simulink model "adapt_mem"  (Simulink 7.9)
settings: Solver=ode45  StartTime=0.0  StopTime=100  RelTol=1e-3
settings Model: Creator=Floater  LastModifiedBy=jdenil
settings OptimizationCC: InlineParams=on  InitFltsAndDblsToZero=on
settings DebuggingCC: FcnCallInpInsideContextMsg=Use local settings  StrictBusMsg=Warning
settings GRTTargetCC: CombineOutputUpdateFcns=off  GRTInterface=on

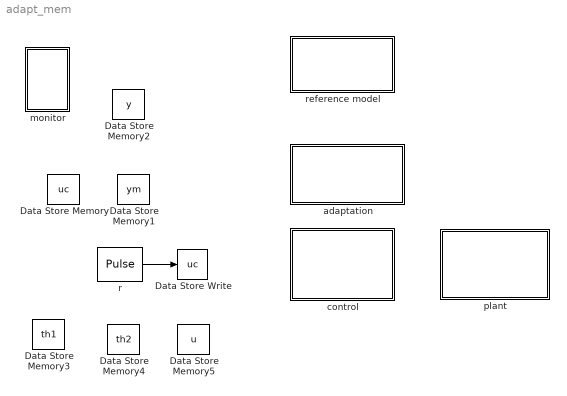
== system adapt_mem ==
  Data Store Memory : DataStoreMemory  DataStoreName=uc  ReadBeforeWriteMsg=warning  WriteAfterWriteMsg=warning  WriteAfterReadMsg=warning
  Data Store Memory1 : DataStoreMemory  DataStoreName=ym  ReadBeforeWriteMsg=warning  WriteAfterWriteMsg=warning  WriteAfterReadMsg=warning
  Data Store Memory2 : DataStoreMemory  DataStoreName=y  ReadBeforeWriteMsg=warning  WriteAfterWriteMsg=warning  WriteAfterReadMsg=warning
  Data Store Memory3 : DataStoreMemory  DataStoreName=th1  ReadBeforeWriteMsg=warning  WriteAfterWriteMsg=warning  WriteAfterReadMsg=warning
  Data Store Memory4 : DataStoreMemory  DataStoreName=th2  ReadBeforeWriteMsg=warning  WriteAfterWriteMsg=warning  WriteAfterReadMsg=warning
  Data Store Memory5 : DataStoreMemory  DataStoreName=u  ReadBeforeWriteMsg=warning  WriteAfterWriteMsg=warning  WriteAfterReadMsg=warning
  Data Store Write : DataStoreWrite  DataStoreName=uc
  adaptation : Subsystem  TreatAsAtomicUnit=on
  control : Subsystem  TreatAsAtomicUnit=on
      settings: AttributesFormatString=%<IsSubsystemVirtual>\n%<TreatAsAtomicUnit>
  monitor : Subsystem  TreatAsAtomicUnit=on
  plant : Subsystem  Priority=1  TreatAsAtomicUnit=on
  r : DiscretePulseGenerator  PulseType=Time based  Period=20  PulseWidth=50
  reference model : Subsystem  TreatAsAtomicUnit=on
      settings: AttributesFormatString=%<Priority>
  wires:
  r/1 -> Data Store Write/1

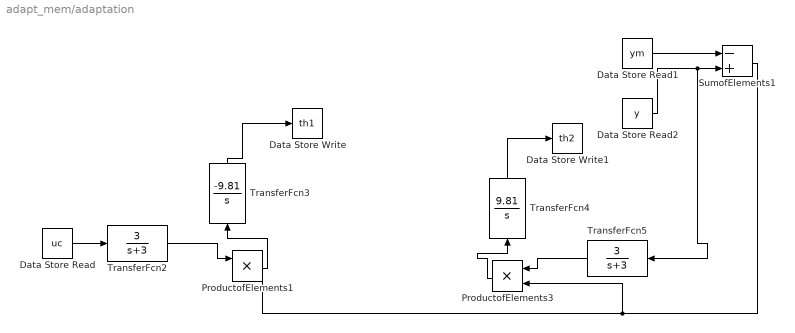
== system adapt_mem/adaptation ==
  Data Store Read : DataStoreRead  DataStoreName=uc
  Data Store Read1 : DataStoreRead  DataStoreName=ym
  Data Store Read2 : DataStoreRead  DataStoreName=y
  Data Store Write : DataStoreWrite  DataStoreName=th1
  Data Store Write1 : DataStoreWrite  DataStoreName=th2
  ProductofElements1 : Product  Inputs=**
  ProductofElements3 : Product  Inputs=**
  SumofElements1 : Sum  Inputs=-+
  TransferFcn2 : TransferFcn  Numerator=[3]  Denominator=[1 3]
  TransferFcn3 : TransferFcn  Numerator=[-9.81]  Denominator=[1 0]
  TransferFcn4 : TransferFcn  Numerator=[9.81]  Denominator=[1 0]
  TransferFcn5 : TransferFcn  Numerator=[3]  Denominator=[1 3]
  wires:
  TransferFcn2/1 -> ProductofElements1/1
  ProductofElements1/1 -> TransferFcn3/1
  TransferFcn3/1 -> Data Store Write/1
  TransferFcn4/1 -> Data Store Write1/1
  ProductofElements3/1 -> TransferFcn4/1
  TransferFcn5/1 -> ProductofElements3/1
  SumofElements1/1 -> ProductofElements1/2, ProductofElements3/2
  Data Store Read2/1 -> SumofElements1/2, TransferFcn5/1
  Data Store Read/1 -> TransferFcn2/1
  Data Store Read1/1 -> SumofElements1/1

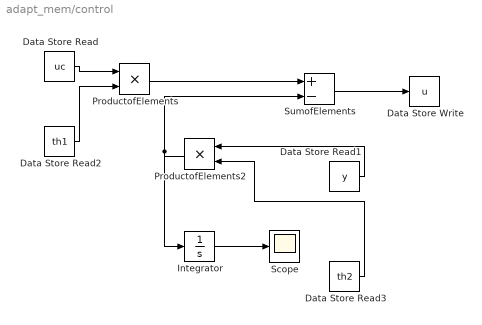
== system adapt_mem/control ==
  Data Store Read : DataStoreRead  DataStoreName=uc
  Data Store Read1 : DataStoreRead  DataStoreName=y
  Data Store Read2 : DataStoreRead  DataStoreName=th1
  Data Store Read3 : DataStoreRead  DataStoreName=th2
  Data Store Write : DataStoreWrite  DataStoreName=u
  Integrator : Integrator
  ProductofElements : Product  Inputs=**
  ProductofElements2 : Product  Inputs=**
  Scope : Scope
      settings: SaveName=ScopeData2
  SumofElements : Sum  Inputs=+-
  wires:
  ProductofElements/1 -> SumofElements/1
  ProductofElements2/1 -> Integrator/1, SumofElements/2
  Data Store Read/1 -> ProductofElements/1
  Data Store Read2/1 -> ProductofElements/2
  Data Store Read1/1 -> ProductofElements2/1
  Data Store Read3/1 -> ProductofElements2/2
  SumofElements/1 -> Data Store Write/1
  Integrator/1 -> Scope/1

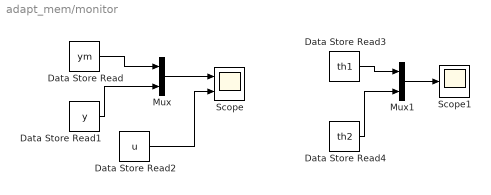
== system adapt_mem/monitor ==
  Data Store Read : DataStoreRead  DataStoreName=ym
  Data Store Read1 : DataStoreRead  DataStoreName=y
  Data Store Read2 : DataStoreRead  DataStoreName=u
  Data Store Read3 : DataStoreRead  DataStoreName=th1
  Data Store Read4 : DataStoreRead  DataStoreName=th2
  Mux : Mux  Inputs=2
  Mux1 : Mux  Inputs=2
  Scope : Scope  NumInputPorts=2
      settings: TimeRange=100  YMin=0~-0.5  YMax=1.4~2.5
  Scope1 : Scope
      settings: TimeRange=100  YMin=-0.5  YMax=3
  wires:
  Mux/1 -> Scope/1
  Mux1/1 -> Scope1/1
  Data Store Read3/1 -> Mux1/1
  Data Store Read4/1 -> Mux1/2
  Data Store Read1/1 -> Mux/2
  Data Store Read2/1 -> Scope/2
  Data Store Read/1 -> Mux/1

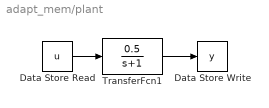
== system adapt_mem/plant ==
  Data Store Read : DataStoreRead  DataStoreName=u
  Data Store Write : DataStoreWrite  DataStoreName=y
  TransferFcn1 : TransferFcn  Numerator=[0.5]  Denominator=[1 1]
  wires:
  Data Store Read/1 -> TransferFcn1/1
  TransferFcn1/1 -> Data Store Write/1

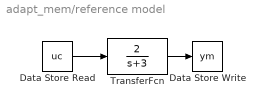
== system adapt_mem/reference model ==
  Data Store Read : DataStoreRead  DataStoreName=uc
  Data Store Write : DataStoreWrite  DataStoreName=ym
  TransferFcn : TransferFcn  Numerator=[2]  Denominator=[1 3]
  wires:
  Data Store Read/1 -> TransferFcn/1
  TransferFcn/1 -> Data Store Write/1
